simulink model "fft_2"  (R2019a)
settings: Solver=VariableStepAuto  StartTime=0.0  StopTime=T-Te  RelTol=1e-3
values from neighbouring files (symbols this model uses):
  den = [1.7483*10.^(-23) 7.6663*10.^(-18) 1.162*10.^(-11) 3.0332*10.^(-6) 1]    [traitementSignal.m]
  F0 = 85000    [traitementSignal.m]
  F1 = 85005.9    [traitementSignal.m]
  F2 = 90000    [traitementSignal.m]
  F3 = 95000    [traitementSignal.m]
  F4 = 100000    [traitementSignal.m]
  F5 = 115000    [traitementSignal.m]
  F6 = 120000    [traitementSignal.m]
  num = 1    [traitementSignal.m]
  Te = 1/Fe    (= 3.125e-06)    [traitementSignal.m]
settings Model: Creator=fleon  LastModifiedBy=fleon

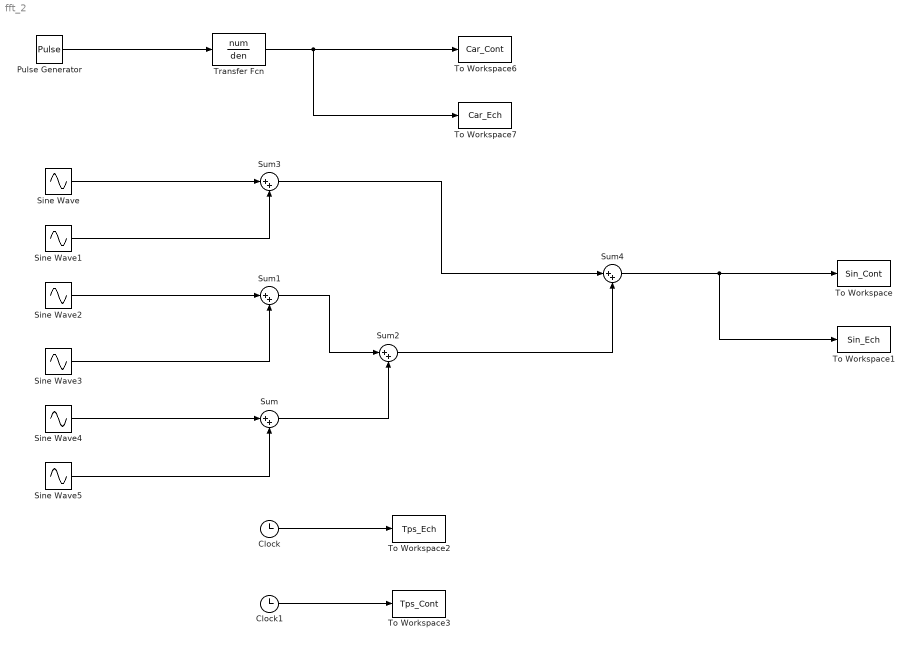
== system fft_2 ==
  Clock : Clock
  Clock1 : Clock
  Pulse Generator : DiscretePulseGenerator  PulseType=Time based  Period=1/F0  PulseWidth=50
  Sine Wave : Sin  Frequency=2*pi*F1  SampleTime=0
  Sine Wave1 : Sin  Frequency=2*pi*F2  SampleTime=0
  Sine Wave2 : Sin  Frequency=2*pi*F3  SampleTime=0
  Sine Wave3 : Sin  Frequency=2*pi*F4  SampleTime=0
  Sine Wave4 : Sin  Frequency=2*pi*F5  SampleTime=0
  Sine Wave5 : Sin  Frequency=2*pi*F6  SampleTime=0
  Sum{,1..4} (5 alike) : Sum  Inputs=|++
  To Workspace : ToWorkspace  VariableName=Sin_Cont  SampleTime=Te/100
  To Workspace1 : ToWorkspace  VariableName=Sin_Ech  SampleTime=Te
  To Workspace2 : ToWorkspace  VariableName=Tps_Ech  SampleTime=Te
  To Workspace3 : ToWorkspace  VariableName=Tps_Cont  SampleTime=Te/100
  To Workspace6 : ToWorkspace  VariableName=Car_Cont  SampleTime=Te/100
  To Workspace7 : ToWorkspace  VariableName=Car_Ech  SampleTime=Te
  Transfer Fcn : TransferFcn  Numerator=num  Denominator=den
  wires:
  Clock1/1 -> To Workspace3/1
  Sine Wave/1 -> Sum3/1
  Clock/1 -> To Workspace2/1
  Sine Wave5/1 -> Sum/2
  Sine Wave4/1 -> Sum/1
  Sine Wave3/1 -> Sum1/2
  Sine Wave2/1 -> Sum1/1
  Sum/1 -> Sum2/2
  Sum1/1 -> Sum2/1
  Sine Wave1/1 -> Sum3/2
  Sum2/1 -> Sum4/2
  Sum3/1 -> Sum4/1
  Sum4/1 -> To Workspace1/1, To Workspace/1
  Pulse Generator/1 -> Transfer Fcn/1
  Transfer Fcn/1 -> To Workspace6/1, To Workspace7/1
